simulink model "carPlant_OMVBandoHFHumanFollower_4"  (R2018b)
settings: Solver=VariableStepAuto  StartTime=0.0  StopTime=100  RelTol=1e-3
libraries: autolibshared x4, vehdynlibsteering x4
settings Model: Creator=ckreienk  LastModifiedBy=ckreienk

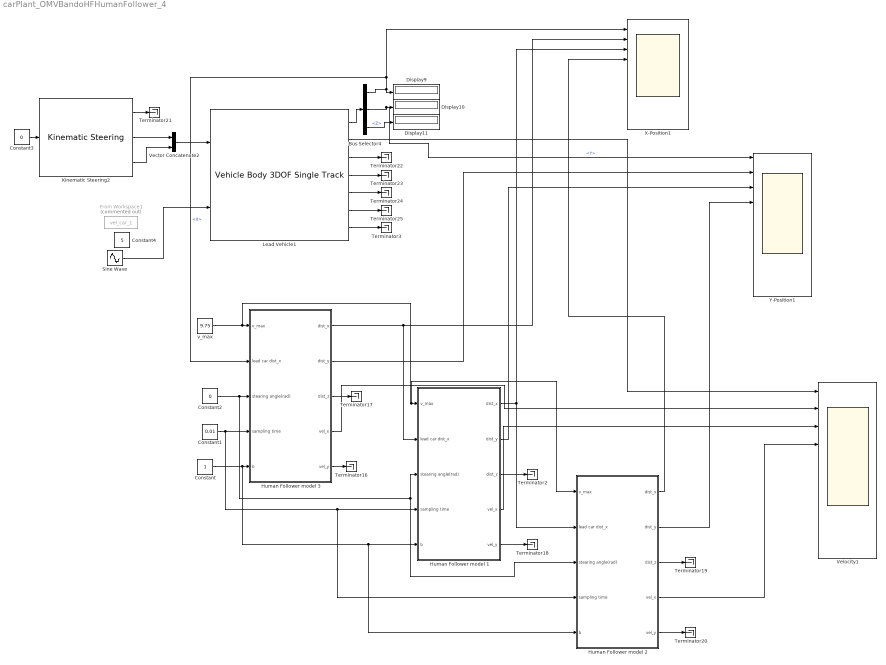
== system carPlant_OMVBandoHFHumanFollower_4 ==
  Bus Selector4 : BusSelector  OutputSignals=InertFrm.Geom.Disp.X,InertFrm.Geom.Disp.Y,InertFrm.Geom.Disp.Z
  Constant : Constant
  Constant1 : Constant  Value=0.01
  Constant2 : Constant  Value=0
  Constant3 : Constant  Value=0
  Constant4 : Constant  Value=5
  Display10 : Display
  Display11 : Display
  Display9 : Display
  From Workspace1 : FromWorkspace  Commented=on  VariableName=vel_car_1  SampleTime=0.1
  Human Follower model 1 : Subsystem
  Human Follower model 2 : Subsystem
  Human Follower model 3 : Subsystem
  Kinematic Steering2 : vehdynlibsteering/Kinematic Steering  StrgType=Rack and pinion  StrgRatioType=Constant  Loc=Front  NrmlFctr=0.01  TrckWdth=1  WhlBase=1.524  Db=0  StrgRng=1.25*pi  StrgAngBpts="[-6.2832   -5.0265   -3.7699   -2.5133   -1.2566         0    1.2566    2.5133    3.7699    5.0265    6.2832]"  StrgRatioTbl=|  StrgRatio=100  StrgArmLngth=0.1  RckCsLngth=0.5  TieRodLngth=0.248  D=0.2  PnnRadius=0.0057  PnnRadiusTbl="[0.0055    0.0055    0.0056    0.0057    0.0058    0.0057    0.0057    0.0057    0.0056    0.0055    0.0055]"  RodLngth=0.1  ParaArmLngth=0.9  aMode=2
      | [13.5000   13.3750   13.2500   13.1250   13.0000   13.0000   13.0000   13.1250   13.2500   13.3750   13.5000
      | ]
      settings: SourceProductName=Vehicle Dynamics Blockset
  Lead Vehicle1 : autolibshared/Vehicle Body 3DOF Single Track  trackMode=Dual  inputMode=External longitudinal velocity  frontSteerMode=on  rearSteerMode=off  windMode=off  muMode=off  extFMode=off  extMMode=off  aMode=2  NF=2  NR=2  m=2000  a=1.4  b=1.6  h=0.35  X_o=40  xdot_o=0  CalphaMode=off  sigmaMode=off  d=0  w=[1.4,1.4]  Cy_f=12e3  Cy_r=11e3  sigma_f=.1  sigma_r=.1  alpha_f_brk=[-.1 .1]  Cy_f_data=[-9e3 9e3]  alpha_r_brk=[-.1 .1]  Cy_r_data=[-9e3 9e3]  Y_o=0  ydot_o=0  Izz=4000  psi_o=0  r_o=0  Af=2  Cd=.3  Cl=.1  Cpm=.1  beta_w=[0:0.01:0.3]  Cs=[0:0.03:0.9]  Cym=[0:0.01:0.3]  Pabs=101325  Tair=273  g=9.81  mu=1  xdot_tol=.01  Fznom=5000  Fxtire_sat=7e4  Fytire_sat=7e4  longOff=0  latOff=0  vertOff=0
      settings: SourceProductName=Powertrain Blockset  SourceProductBaseCode=PW
  Sine Wave : Sin  Amplitude=5  Frequency=0.05  SampleTime=0
  Terminator{2..3,16..25} (12 alike) : Terminator
  Vector Concatenate2 : Concatenate
  Velocity1 : Scope  NumInputPorts=10
  X-Position1 : Scope  NumInputPorts=10
  Y-Position1 : Scope  NumInputPorts=10
  "v_max " : Constant  Value=9.75
  wires:
  Bus Selector4/3 -> Display11/1  "<Z>"
  Lead Vehicle1/3 -> Terminator22/1
  Human Follower model 3/5(vel_y) -> Terminator16/1
  Kinematic Steering2/1 -> Terminator21/1
  Bus Selector4/2 -> Display10/1, Y-Position1/1  "<Y>"
  Lead Vehicle1/7 -> Terminator3/1
  Kinematic Steering2/3 -> Vector Concatenate2/2
  Bus Selector4/1 -> Human Follower model 3/2(lead car dist_x), X-Position1/1, Display9/1  "<X>"
  Lead Vehicle1/6 -> Terminator25/1
  Lead Vehicle1/1 -> Bus Selector4/1
  Constant3/1 -> Kinematic Steering2/1
  Human Follower model 2/5(vel_y) -> Terminator20/1
  Lead Vehicle1/4 -> Terminator23/1
  Human Follower model 1/5(vel_y) -> Terminator18/1
  Human Follower model 2/3(dist_z) -> Terminator19/1
  Vector Concatenate2/1 -> Lead Vehicle1/1
  Lead Vehicle1/5 -> Terminator24/1
  Kinematic Steering2/2 -> Vector Concatenate2/1
  Human Follower model 3/3(dist_z) -> Terminator17/1
  Human Follower model 1/3(dist_z) -> Terminator2/1
  "v_max "/1 -> Human Follower model 2/1(v_max), Human Follower model 1/1(v_max), Human Follower model 3/1(v_max)
  Constant2/1 -> Human Follower model 3/3(stearing angle(rad)), Human Follower model 2/3(stearing angle(rad)), Human Follower model 1/3(stearing angle(rad))
  Constant1/1 -> Human Follower model 3/4(sampling time), Human Follower model 1/4(sampling time), Human Follower model 2/4(sampling time)
  Constant/1 -> Human Follower model 1/5(b), Human Follower model 2/5(b), Human Follower model 3/5(b)
  Human Follower model 3/1(dist_x) -> X-Position1/2, Human Follower model 1/2(lead car dist_x)
  Human Follower model 1/1(dist_x) -> Human Follower model 2/2(lead car dist_x), X-Position1/3
  Human Follower model 2/1(dist_x) -> X-Position1/4
  Human Follower model 3/2(dist_y) -> Y-Position1/2
  Human Follower model 1/2(dist_y) -> Y-Position1/3
  Human Follower model 2/2(dist_y) -> Y-Position1/4
  Human Follower model 3/4(vel_x) -> Velocity1/2
  Human Follower model 1/4(vel_x) -> Velocity1/3
  Human Follower model 2/4(vel_x) -> Velocity1/4
  Lead Vehicle1/2 -> Velocity1/1
  Sine Wave/1 -> Lead Vehicle1/2

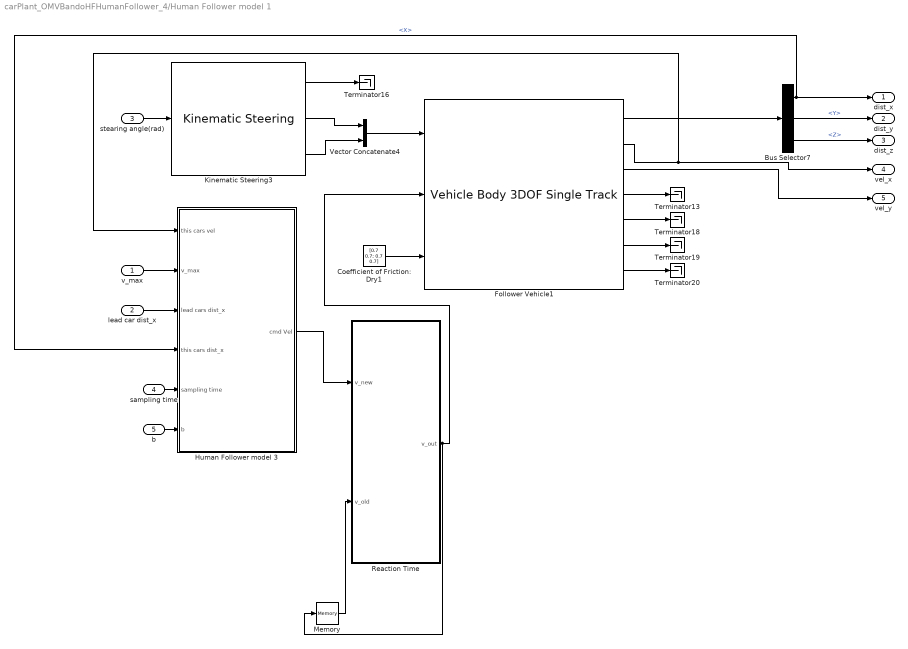
== system carPlant_OMVBandoHFHumanFollower_4/Human Follower model 1 ==
  v_max : Inport
  lead car dist_x : Inport  Port=2
  stearing angle(rad) : Inport  Port=3
  sampling time : Inport  Port=4
  b : Inport  Port=5
  Bus Selector7 : BusSelector  OutputSignals=InertFrm.Cg.Disp.X,InertFrm.Cg.Disp.Y,InertFrm.Cg.Disp.Z
  Coefficient of Friction: Dry1 : Constant  Value=[0.7 0.7; 0.7 0.7]
  Follower Vehicle1 : autolibshared/Vehicle Body 3DOF Single Track  trackMode=Dual  inputMode=External longitudinal velocity  frontSteerMode=on  rearSteerMode=off  windMode=off  muMode=on  extFMode=off  extMMode=off  aMode=2  NF=2  NR=2  m=2000  a=1.4  b=1.6  h=0.35  X_o=20  xdot_o=0  CalphaMode=off  sigmaMode=on  d=0  w=[1.4,1.4]  Cy_f=12e3  Cy_r=11e3  sigma_f=.1  sigma_r=.1  alpha_f_brk=[-.1 .1]  Cy_f_data=[-9e3 9e3]  alpha_r_brk=[-.1 .1]  Cy_r_data=[-9e3 9e3]  Y_o=0  ydot_o=0  Izz=4000  psi_o=0  r_o=0  Af=2  Cd=.3  Cl=.1  Cpm=.1  beta_w=[0:0.01:0.3]  Cs=[0:0.03:0.9]  Cym=[0:0.01:0.3]  Pabs=101325  Tair=273  g=9.81  mu=1  xdot_tol=.01  Fznom=5000  Fxtire_sat=7e4  Fytire_sat=7e4  longOff=0  latOff=0  vertOff=0
      settings: SourceProductName=Powertrain Blockset  SourceProductBaseCode=PW
  Human Follower model 3 : Subsystem
  Kinematic Steering3 : vehdynlibsteering/Kinematic Steering  StrgType=Ackerman  StrgRatioType=Constant  Loc=Front  NrmlFctr=0.01  TrckWdth=1  WhlBase=1.524  Db=0  StrgRng=1.25*pi  StrgAngBpts="[-6.2832   -5.0265   -3.7699   -2.5133   -1.2566         0    1.2566    2.5133    3.7699    5.0265    6.2832]"  StrgRatioTbl=|  StrgRatio=100  StrgArmLngth=0.1  RckCsLngth=0.5  TieRodLngth=0.248  D=0.2  PnnRadius=0.0057  PnnRadiusTbl="[0.0055    0.0055    0.0056    0.0057    0.0058    0.0057    0.0057    0.0057    0.0056    0.0055    0.0055]"  RodLngth=0.1  ParaArmLngth=0.9  aMode=2
      | [13.5000   13.3750   13.2500   13.1250   13.0000   13.0000   13.0000   13.1250   13.2500   13.3750   13.5000
      | ]
      settings: SourceProductName=Vehicle Dynamics Blockset
  Memory : Memory
  Reaction Time : Subsystem
  Terminator{13,16,18..20} (5 alike) : Terminator
  Vector Concatenate4 : Concatenate
  dist_x : Outport
  dist_y : Outport  Port=2
  dist_z : Outport  Port=3
  vel_x : Outport  Port=4
  vel_y : Outport  Port=5
  wires:
  Coefficient of Friction: Dry1/1 -> Follower Vehicle1/3
  Kinematic Steering3/3 -> Vector Concatenate4/2
  stearing angle(rad)/1 -> Kinematic Steering3/1
  Kinematic Steering3/2 -> Vector Concatenate4/1
  Bus Selector7/2 -> dist_y/1  "<Y>"
  Kinematic Steering3/1 -> Terminator16/1
  Follower Vehicle1/1 -> Bus Selector7/1
  Vector Concatenate4/1 -> Follower Vehicle1/1
  Follower Vehicle1/7 -> Terminator20/1
  Follower Vehicle1/3 -> vel_y/1
  Follower Vehicle1/4 -> Terminator13/1
  Bus Selector7/1 -> Human Follower model 3/4(this cars dist_x), dist_x/1  "<X>"
  Follower Vehicle1/6 -> Terminator19/1
  Follower Vehicle1/5 -> Terminator18/1
  Bus Selector7/3 -> dist_z/1  "<Z>"
  sampling time/1 -> Human Follower model 3/5(sampling time)
  b/1 -> Human Follower model 3/6(b)
  lead car dist_x/1 -> Human Follower model 3/3(lead cars dist_x)
  v_max/1 -> Human Follower model 3/2(v_max)
  Follower Vehicle1/2 -> Human Follower model 3/1(this cars vel), vel_x/1
  Human Follower model 3/1(cmd Vel) -> Reaction Time/1(v_new)
  Reaction Time/1(v_out) -> Memory/1, Follower Vehicle1/2
  Memory/1 -> Reaction Time/2(v_old)

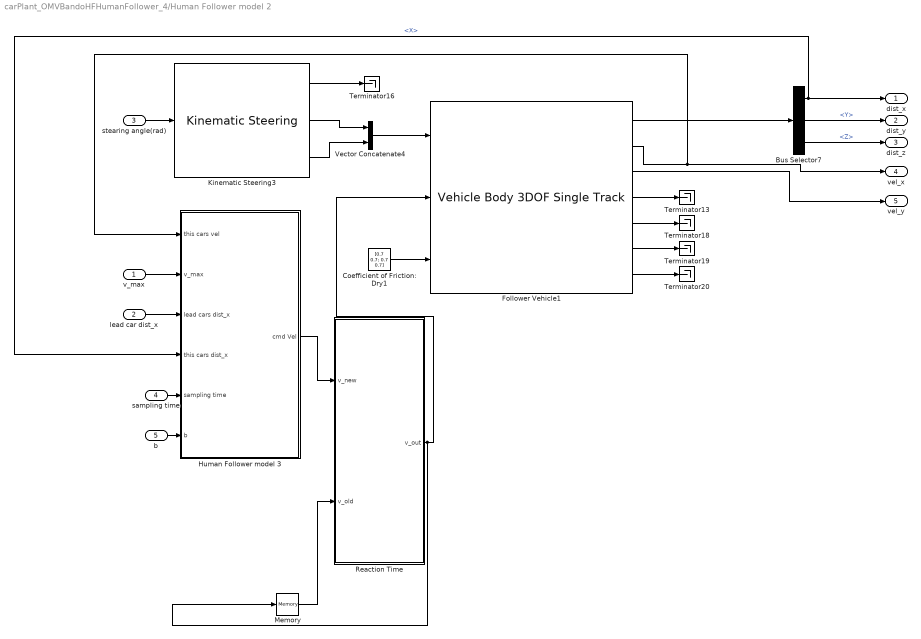
== system carPlant_OMVBandoHFHumanFollower_4/Human Follower model 2 ==
  v_max : Inport
  lead car dist_x : Inport  Port=2
  stearing angle(rad) : Inport  Port=3
  sampling time : Inport  Port=4
  b : Inport  Port=5
  Bus Selector7 : BusSelector  OutputSignals=InertFrm.Cg.Disp.X,InertFrm.Cg.Disp.Y,InertFrm.Cg.Disp.Z
  Coefficient of Friction: Dry1 : Constant  Value=[0.7 0.7; 0.7 0.7]
  Follower Vehicle1 : autolibshared/Vehicle Body 3DOF Single Track  trackMode=Dual  inputMode=External longitudinal velocity  frontSteerMode=on  rearSteerMode=off  windMode=off  muMode=on  extFMode=off  extMMode=off  aMode=2  NF=2  NR=2  m=2000  a=1.4  b=1.6  h=0.35  X_o=10  xdot_o=0  CalphaMode=off  sigmaMode=on  d=0  w=[1.4,1.4]  Cy_f=12e3  Cy_r=11e3  sigma_f=.1  sigma_r=.1  alpha_f_brk=[-.1 .1]  Cy_f_data=[-9e3 9e3]  alpha_r_brk=[-.1 .1]  Cy_r_data=[-9e3 9e3]  Y_o=0  ydot_o=0  Izz=4000  psi_o=0  r_o=0  Af=2  Cd=.3  Cl=.1  Cpm=.1  beta_w=[0:0.01:0.3]  Cs=[0:0.03:0.9]  Cym=[0:0.01:0.3]  Pabs=101325  Tair=273  g=9.81  mu=1  xdot_tol=.01  Fznom=5000  Fxtire_sat=7e4  Fytire_sat=7e4  longOff=0  latOff=0  vertOff=0
      settings: SourceProductName=Powertrain Blockset  SourceProductBaseCode=PW
  Human Follower model 3 : Subsystem
  Kinematic Steering3 : vehdynlibsteering/Kinematic Steering  StrgType=Ackerman  StrgRatioType=Constant  Loc=Front  NrmlFctr=0.01  TrckWdth=1  WhlBase=1.524  Db=0  StrgRng=1.25*pi  StrgAngBpts="[-6.2832   -5.0265   -3.7699   -2.5133   -1.2566         0    1.2566    2.5133    3.7699    5.0265    6.2832]"  StrgRatioTbl=|  StrgRatio=100  StrgArmLngth=0.1  RckCsLngth=0.5  TieRodLngth=0.248  D=0.2  PnnRadius=0.0057  PnnRadiusTbl="[0.0055    0.0055    0.0056    0.0057    0.0058    0.0057    0.0057    0.0057    0.0056    0.0055    0.0055]"  RodLngth=0.1  ParaArmLngth=0.9  aMode=2
      | [13.5000   13.3750   13.2500   13.1250   13.0000   13.0000   13.0000   13.1250   13.2500   13.3750   13.5000
      | ]
      settings: SourceProductName=Vehicle Dynamics Blockset
  Memory : Memory
  Reaction Time : Subsystem
  Terminator{13,16,18..20} (5 alike) : Terminator
  Vector Concatenate4 : Concatenate
  dist_x : Outport
  dist_y : Outport  Port=2
  dist_z : Outport  Port=3
  vel_x : Outport  Port=4
  vel_y : Outport  Port=5
  wires:
  Coefficient of Friction: Dry1/1 -> Follower Vehicle1/3
  Kinematic Steering3/3 -> Vector Concatenate4/2
  stearing angle(rad)/1 -> Kinematic Steering3/1
  Kinematic Steering3/2 -> Vector Concatenate4/1
  Bus Selector7/2 -> dist_y/1  "<Y>"
  Kinematic Steering3/1 -> Terminator16/1
  Follower Vehicle1/1 -> Bus Selector7/1
  Vector Concatenate4/1 -> Follower Vehicle1/1
  Follower Vehicle1/7 -> Terminator20/1
  Follower Vehicle1/3 -> vel_y/1
  Follower Vehicle1/4 -> Terminator13/1
  Bus Selector7/1 -> Human Follower model 3/4(this cars dist_x), dist_x/1  "<X>"
  Follower Vehicle1/6 -> Terminator19/1
  Follower Vehicle1/5 -> Terminator18/1
  Bus Selector7/3 -> dist_z/1  "<Z>"
  sampling time/1 -> Human Follower model 3/5(sampling time)
  b/1 -> Human Follower model 3/6(b)
  lead car dist_x/1 -> Human Follower model 3/3(lead cars dist_x)
  v_max/1 -> Human Follower model 3/2(v_max)
  Follower Vehicle1/2 -> Human Follower model 3/1(this cars vel), vel_x/1
  Reaction Time/1(v_out) -> Memory/1, Follower Vehicle1/2
  Human Follower model 3/1(cmd Vel) -> Reaction Time/1(v_new)
  Memory/1 -> Reaction Time/2(v_old)

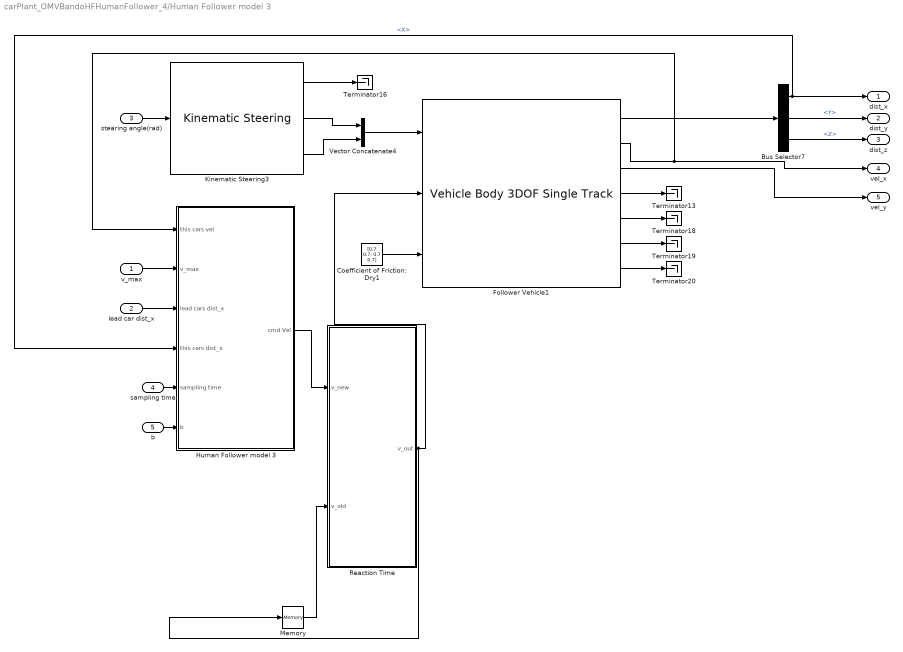
== system carPlant_OMVBandoHFHumanFollower_4/Human Follower model 3 ==
  v_max : Inport
  lead car dist_x : Inport  Port=2
  stearing angle(rad) : Inport  Port=3
  sampling time : Inport  Port=4
  b : Inport  Port=5
  Bus Selector7 : BusSelector  OutputSignals=InertFrm.Cg.Disp.X,InertFrm.Cg.Disp.Y,InertFrm.Cg.Disp.Z
  Coefficient of Friction: Dry1 : Constant  Value=[0.7 0.7; 0.7 0.7]
  Follower Vehicle1 : autolibshared/Vehicle Body 3DOF Single Track  trackMode=Dual  inputMode=External longitudinal velocity  frontSteerMode=on  rearSteerMode=off  windMode=off  muMode=on  extFMode=off  extMMode=off  aMode=2  NF=2  NR=2  m=2000  a=1.4  b=1.6  h=0.35  X_o=30  xdot_o=0  CalphaMode=off  sigmaMode=on  d=0  w=[1.4,1.4]  Cy_f=12e3  Cy_r=11e3  sigma_f=.1  sigma_r=.1  alpha_f_brk=[-.1 .1]  Cy_f_data=[-9e3 9e3]  alpha_r_brk=[-.1 .1]  Cy_r_data=[-9e3 9e3]  Y_o=0  ydot_o=0  Izz=4000  psi_o=0  r_o=0  Af=2  Cd=.3  Cl=.1  Cpm=.1  beta_w=[0:0.01:0.3]  Cs=[0:0.03:0.9]  Cym=[0:0.01:0.3]  Pabs=101325  Tair=273  g=9.81  mu=1  xdot_tol=.01  Fznom=5000  Fxtire_sat=7e4  Fytire_sat=7e4  longOff=0  latOff=0  vertOff=0
      settings: SourceProductName=Powertrain Blockset  SourceProductBaseCode=PW
  Human Follower model 3 : Subsystem
  Kinematic Steering3 : vehdynlibsteering/Kinematic Steering  StrgType=Ackerman  StrgRatioType=Constant  Loc=Front  NrmlFctr=0.01  TrckWdth=1  WhlBase=1.524  Db=0  StrgRng=1.25*pi  StrgAngBpts="[-6.2832   -5.0265   -3.7699   -2.5133   -1.2566         0    1.2566    2.5133    3.7699    5.0265    6.2832]"  StrgRatioTbl=|  StrgRatio=100  StrgArmLngth=0.1  RckCsLngth=0.5  TieRodLngth=0.248  D=0.2  PnnRadius=0.0057  PnnRadiusTbl="[0.0055    0.0055    0.0056    0.0057    0.0058    0.0057    0.0057    0.0057    0.0056    0.0055    0.0055]"  RodLngth=0.1  ParaArmLngth=0.9  aMode=2
      | [13.5000   13.3750   13.2500   13.1250   13.0000   13.0000   13.0000   13.1250   13.2500   13.3750   13.5000
      | ]
      settings: SourceProductName=Vehicle Dynamics Blockset
  Memory : Memory
  Reaction Time : Subsystem
  Terminator{13,16,18..20} (5 alike) : Terminator
  Vector Concatenate4 : Concatenate
  dist_x : Outport
  dist_y : Outport  Port=2
  dist_z : Outport  Port=3
  vel_x : Outport  Port=4
  vel_y : Outport  Port=5
  wires:
  Coefficient of Friction: Dry1/1 -> Follower Vehicle1/3
  Kinematic Steering3/3 -> Vector Concatenate4/2
  stearing angle(rad)/1 -> Kinematic Steering3/1
  Kinematic Steering3/2 -> Vector Concatenate4/1
  Bus Selector7/2 -> dist_y/1  "<Y>"
  Kinematic Steering3/1 -> Terminator16/1
  Follower Vehicle1/1 -> Bus Selector7/1
  Vector Concatenate4/1 -> Follower Vehicle1/1
  Follower Vehicle1/7 -> Terminator20/1
  Follower Vehicle1/3 -> vel_y/1
  Follower Vehicle1/4 -> Terminator13/1
  Bus Selector7/1 -> Human Follower model 3/4(this cars dist_x), dist_x/1  "<X>"
  Follower Vehicle1/6 -> Terminator19/1
  Follower Vehicle1/5 -> Terminator18/1
  Bus Selector7/3 -> dist_z/1  "<Z>"
  sampling time/1 -> Human Follower model 3/5(sampling time)
  b/1 -> Human Follower model 3/6(b)
  lead car dist_x/1 -> Human Follower model 3/3(lead cars dist_x)
  v_max/1 -> Human Follower model 3/2(v_max)
  Follower Vehicle1/2 -> Human Follower model 3/1(this cars vel), vel_x/1
  Human Follower model 3/1(cmd Vel) -> Reaction Time/1(v_new)
  Reaction Time/1(v_out) -> Memory/1, Follower Vehicle1/2
  Memory/1 -> Reaction Time/2(v_old)

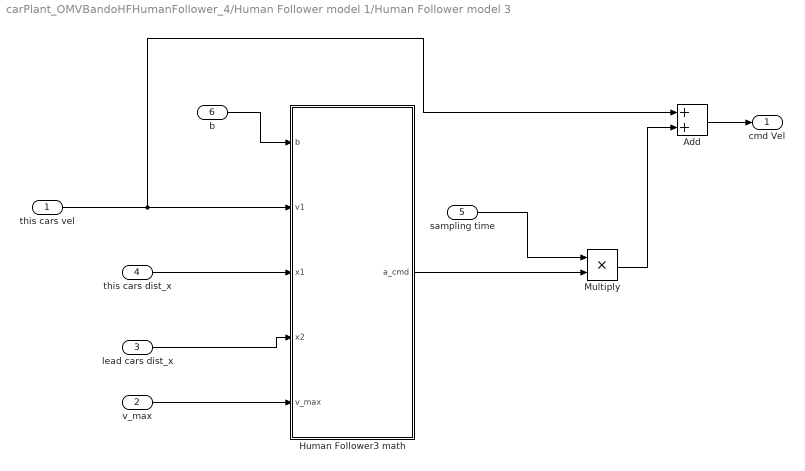
== system carPlant_OMVBandoHFHumanFollower_4/Human Follower model 1/Human Follower model 3 ==
  this cars vel : Inport
  v_max : Inport  Port=2
  lead cars dist_x : Inport  Port=3
  this cars dist_x : Inport  Port=4
  sampling time : Inport  Port=5
  b : Inport  Port=6
  Add : Sum
  Human Follower3 math : Subsystem
  Multiply : Product
  cmd Vel : Outport
  wires:
  sampling time/1 -> Multiply/1
  Multiply/1 -> Add/2
  Human Follower3 math/1(a_cmd) -> Multiply/2
  this cars vel/1 -> Human Follower3 math/2(v1), Add/1
  Add/1 -> cmd Vel/1
  b/1 -> Human Follower3 math/1(b)
  lead cars dist_x/1 -> Human Follower3 math/4(x2)
  v_max/1 -> Human Follower3 math/5(v_max)
  this cars dist_x/1 -> Human Follower3 math/3(x1)

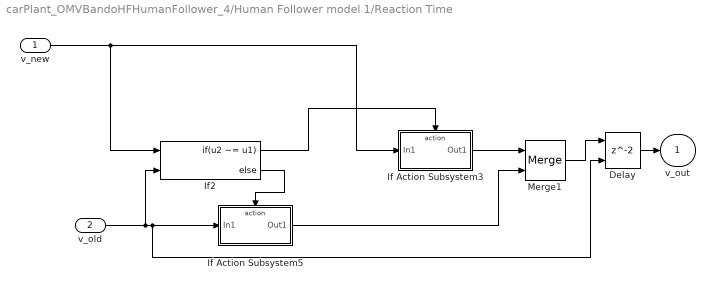
== system carPlant_OMVBandoHFHumanFollower_4/Human Follower model 1/Reaction Time ==
  v_new : Inport
  v_old : Inport  Port=2
  Delay : Delay  InitialConditionSource=Input port
      settings: InputPortMap=u0,p4
  If Action Subsystem3 : Subsystem  TreatAsAtomicUnit=on
  If Action Subsystem5 : Subsystem  TreatAsAtomicUnit=on
  If2 : If  NumInputs=2  IfExpression=u2 ~= u1
  Merge1 : Merge
  v_out : Outport
  wires:
  If Action Subsystem5/1(Out1) -> Merge1/2
  If2/1 -> If Action Subsystem3/Action
  If2/2 -> If Action Subsystem5/Action
  If Action Subsystem3/1(Out1) -> Merge1/1
  v_new/1 -> If2/1, If Action Subsystem3/1(In1)
  Merge1/1 -> Delay/1
  Delay/1 -> v_out/1
  v_old/1 -> If2/2, Delay/2, If Action Subsystem5/1(In1)

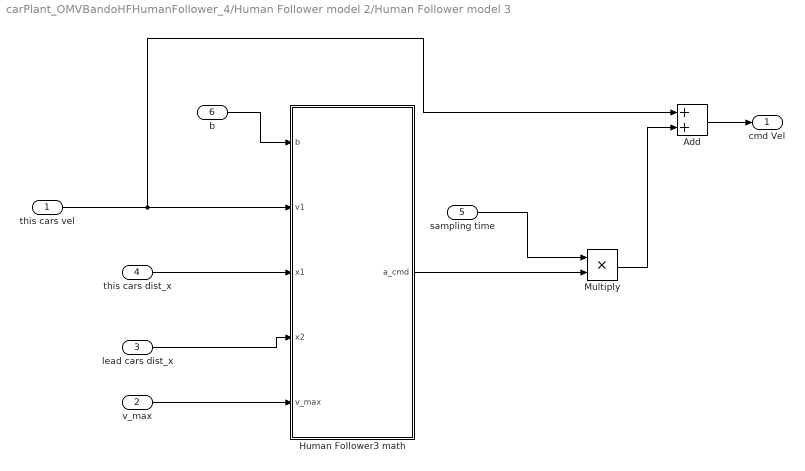
== system carPlant_OMVBandoHFHumanFollower_4/Human Follower model 2/Human Follower model 3 ==
  this cars vel : Inport
  v_max : Inport  Port=2
  lead cars dist_x : Inport  Port=3
  this cars dist_x : Inport  Port=4
  sampling time : Inport  Port=5
  b : Inport  Port=6
  Add : Sum
  Human Follower3 math : Subsystem
  Multiply : Product
  cmd Vel : Outport
  wires:
  sampling time/1 -> Multiply/1
  Multiply/1 -> Add/2
  Human Follower3 math/1(a_cmd) -> Multiply/2
  this cars vel/1 -> Human Follower3 math/2(v1), Add/1
  Add/1 -> cmd Vel/1
  b/1 -> Human Follower3 math/1(b)
  lead cars dist_x/1 -> Human Follower3 math/4(x2)
  v_max/1 -> Human Follower3 math/5(v_max)
  this cars dist_x/1 -> Human Follower3 math/3(x1)

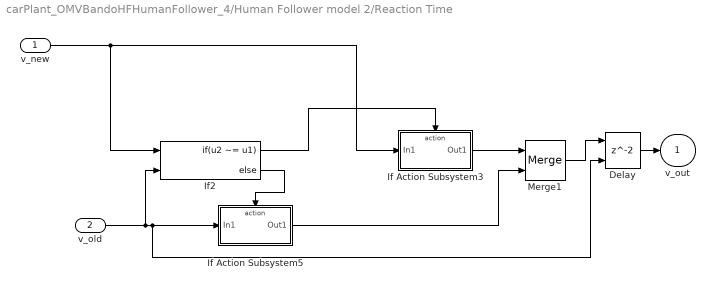
== system carPlant_OMVBandoHFHumanFollower_4/Human Follower model 2/Reaction Time ==
  v_new : Inport
  v_old : Inport  Port=2
  Delay : Delay  InitialConditionSource=Input port
      settings: InputPortMap=u0,p4
  If Action Subsystem3 : Subsystem  TreatAsAtomicUnit=on
  If Action Subsystem5 : Subsystem  TreatAsAtomicUnit=on
  If2 : If  NumInputs=2  IfExpression=u2 ~= u1
  Merge1 : Merge
  v_out : Outport
  wires:
  If Action Subsystem5/1(Out1) -> Merge1/2
  If2/1 -> If Action Subsystem3/Action
  If2/2 -> If Action Subsystem5/Action
  If Action Subsystem3/1(Out1) -> Merge1/1
  v_new/1 -> If2/1, If Action Subsystem3/1(In1)
  Merge1/1 -> Delay/1
  Delay/1 -> v_out/1
  v_old/1 -> If2/2, Delay/2, If Action Subsystem5/1(In1)

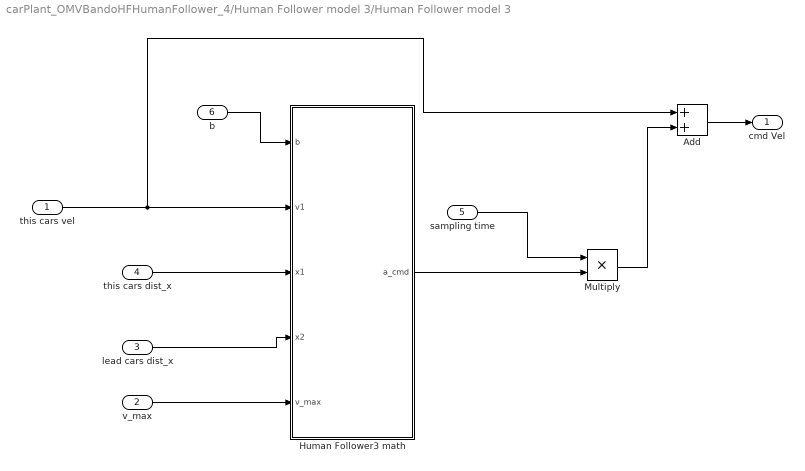
== system carPlant_OMVBandoHFHumanFollower_4/Human Follower model 3/Human Follower model 3 ==
  this cars vel : Inport
  v_max : Inport  Port=2
  lead cars dist_x : Inport  Port=3
  this cars dist_x : Inport  Port=4
  sampling time : Inport  Port=5
  b : Inport  Port=6
  Add : Sum
  Human Follower3 math : Subsystem
  Multiply : Product
  cmd Vel : Outport
  wires:
  sampling time/1 -> Multiply/1
  Multiply/1 -> Add/2
  Human Follower3 math/1(a_cmd) -> Multiply/2
  this cars vel/1 -> Human Follower3 math/2(v1), Add/1
  Add/1 -> cmd Vel/1
  b/1 -> Human Follower3 math/1(b)
  lead cars dist_x/1 -> Human Follower3 math/4(x2)
  v_max/1 -> Human Follower3 math/5(v_max)
  this cars dist_x/1 -> Human Follower3 math/3(x1)

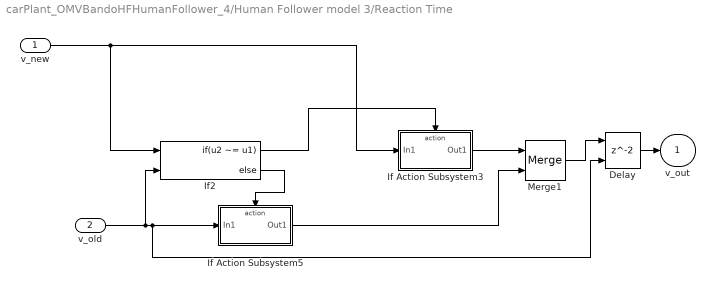
== system carPlant_OMVBandoHFHumanFollower_4/Human Follower model 3/Reaction Time ==
  v_new : Inport
  v_old : Inport  Port=2
  Delay : Delay  InitialConditionSource=Input port
      settings: InputPortMap=u0,p4
  If Action Subsystem3 : Subsystem  TreatAsAtomicUnit=on
  If Action Subsystem5 : Subsystem  TreatAsAtomicUnit=on
  If2 : If  NumInputs=2  IfExpression=u2 ~= u1
  Merge1 : Merge
  v_out : Outport
  wires:
  If Action Subsystem5/1(Out1) -> Merge1/2
  If2/1 -> If Action Subsystem3/Action
  If2/2 -> If Action Subsystem5/Action
  If Action Subsystem3/1(Out1) -> Merge1/1
  v_new/1 -> If2/1, If Action Subsystem3/1(In1)
  Merge1/1 -> Delay/1
  Delay/1 -> v_out/1
  v_old/1 -> If2/2, Delay/2, If Action Subsystem5/1(In1)

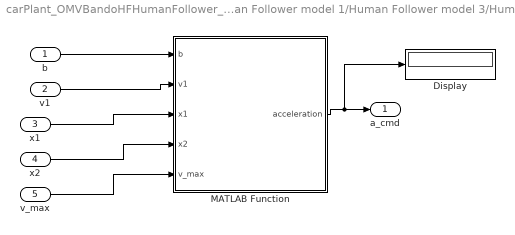
== system carPlant_OMVBandoHFHumanFollower_4/Human Follower model 1/Human Follower model 3/Human Follower3 math ==
  b : Inport
  v1 : Inport  Port=2
  x1 : Inport  Port=3
  x2 : Inport  Port=4
  v_max : Inport  Port=5
  Display : Display
  MATLAB Function : MATLAB Function  TreatAsAtomicUnit=on
  a_cmd : Outport
  wires:
  v1/1 -> MATLAB Function/2(v1)
  b/1 -> MATLAB Function/1(b)
  MATLAB Function/1(acceleration) -> Display/1, a_cmd/1
  x1/1 -> MATLAB Function/3(x1)
  x2/1 -> MATLAB Function/4(x2)
  v_max/1 -> MATLAB Function/5(v_max)

== system carPlant_OMVBandoHFHumanFollower_4/Human Follower model 1/Reaction Time/If Action Subsystem3 ==
  In1 : Inport
  Action Port : ActionPort  ActionType=then
  Out1 : Outport
  wires:
  In1/1 -> Out1/1

== system carPlant_OMVBandoHFHumanFollower_4/Human Follower model 1/Reaction Time/If Action Subsystem5 ==
  In1 : Inport
  Action Port : ActionPort  ActionType=else
  Out1 : Outport
  wires:
  In1/1 -> Out1/1

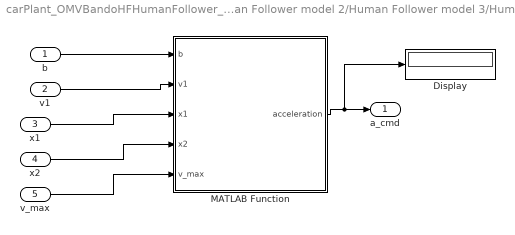
== system carPlant_OMVBandoHFHumanFollower_4/Human Follower model 2/Human Follower model 3/Human Follower3 math ==
  b : Inport
  v1 : Inport  Port=2
  x1 : Inport  Port=3
  x2 : Inport  Port=4
  v_max : Inport  Port=5
  Display : Display
  MATLAB Function : MATLAB Function  TreatAsAtomicUnit=on
  a_cmd : Outport
  wires:
  v1/1 -> MATLAB Function/2(v1)
  b/1 -> MATLAB Function/1(b)
  MATLAB Function/1(acceleration) -> Display/1, a_cmd/1
  x1/1 -> MATLAB Function/3(x1)
  x2/1 -> MATLAB Function/4(x2)
  v_max/1 -> MATLAB Function/5(v_max)

== system carPlant_OMVBandoHFHumanFollower_4/Human Follower model 2/Reaction Time/If Action Subsystem3 ==
  In1 : Inport
  Action Port : ActionPort  ActionType=then
  Out1 : Outport
  wires:
  In1/1 -> Out1/1

== system carPlant_OMVBandoHFHumanFollower_4/Human Follower model 2/Reaction Time/If Action Subsystem5 ==
  In1 : Inport
  Action Port : ActionPort  ActionType=else
  Out1 : Outport
  wires:
  In1/1 -> Out1/1

== system carPlant_OMVBandoHFHumanFollower_4/Human Follower model 3/Human Follower model 3/Human Follower3 math ==
  b : Inport
  v1 : Inport  Port=2
  x1 : Inport  Port=3
  x2 : Inport  Port=4
  v_max : Inport  Port=5
  Display : Display
  MATLAB Function : MATLAB Function  TreatAsAtomicUnit=on
  a_cmd : Outport
  wires:
  v1/1 -> MATLAB Function/2(v1)
  b/1 -> MATLAB Function/1(b)
  MATLAB Function/1(acceleration) -> Display/1, a_cmd/1
  x1/1 -> MATLAB Function/3(x1)
  x2/1 -> MATLAB Function/4(x2)
  v_max/1 -> MATLAB Function/5(v_max)

== system carPlant_OMVBandoHFHumanFollower_4/Human Follower model 3/Reaction Time/If Action Subsystem3 ==
  In1 : Inport
  Action Port : ActionPort  ActionType=then
  Out1 : Outport
  wires:
  In1/1 -> Out1/1

== system carPlant_OMVBandoHFHumanFollower_4/Human Follower model 3/Reaction Time/If Action Subsystem5 ==
  In1 : Inport
  Action Port : ActionPort  ActionType=else
  Out1 : Outport
  wires:
  In1/1 -> Out1/1

== matlab function carPlant_OMVBandoHFHumanFollower_4/Human Follower model 1/Human Follower model 3/Human Follower3 math/MATLAB Function ==
  data: b input; v1 input; x1 input; acceleration output; x2 input; v_max input
function acceleration = fcn(b, v1, x1, x2, v_max)

ds = 2;
L = 4.5;

if x2 == 0
    x2 = 0.1;
end

dx = x2 - x1;

Vd = v_max*(tanh(dx - L - ds) + tanh(L + ds))/(1 + tanh(L + ds));


acceleration = b*(Vd - v1);

== matlab function carPlant_OMVBandoHFHumanFollower_4/Human Follower model 2/Human Follower model 3/Human Follower3 math/MATLAB Function ==
  data: b input; v1 input; x1 input; acceleration output; x2 input; v_max input
function acceleration = fcn(b, v1, x1, x2, v_max)

ds = 2;
L = 4.5;

if x2 == 0
    x2 = 0.1;
end

dx = x2 - x1;

Vd = v_max*(tanh(dx - L - ds) + tanh(L + ds))/(1 + tanh(L + ds));


acceleration = b*(Vd - v1);

== matlab function carPlant_OMVBandoHFHumanFollower_4/Human Follower model 3/Human Follower model 3/Human Follower3 math/MATLAB Function ==
  data: b input; v1 input; x1 input; acceleration output; x2 input; v_max input
function acceleration = fcn(b, v1, x1, x2, v_max)

ds = 2;
L = 4.5;

if x2 == 0
    x2 = 0.1;
end

dx = x2 - x1;

Vd = v_max*(tanh(dx - L - ds) + tanh(L + ds))/(1 + tanh(L + ds));


acceleration = b*(Vd - v1);
